simulink model "APP_Coherency_System_Rev_0_App"  (R2022b)
settings: Solver=FixedStepDiscrete  StartTime=0.0  StopTime=1  FixedStep=1e-3  MaxStep=1e-3  RelTol=1e-3
libraries: simulink x2, pil_lib x1
settings Model: Creator=HiTech  LastModifiedBy=HiTech
settings OptimizationCC: DefaultParameterBehavior=Inlined  UseDivisionForNetSlopeComputation=on  GainParamInheritBuiltInType=on  UseFloatMulNetSlope=on  InlineInvariantSignals=on  PassReuseOutputArgsAs=Individual arguments  ZeroExternalMemoryAtStartup=off  ZeroInternalMemoryAtStartup=off  NoFixptDivByZeroProtection=on  EfficientFloat2IntCast=on  LifeSpan=1  OptimizeBlockOrder=speed  DifferentSizesBufferReuse=on  EfficientTunableParamExpr=on
settings DebuggingCC: ParameterTunabilityLossMsg=error
settings HardwareCC: ProdBitPerPointer=32  ProdBitPerSizeT=32  ProdBitPerPtrDiffT=32  ProdLargestAtomicFloat=None  ProdWordSize=32  ProdLongLongMode=on  ProdHWDeviceType=Atmel->AVR (32-bit)
settings SFSimCC: MATLABDynamicMemAlloc=off
settings RTWCC: Description=Embedded Coder  SystemTargetFile=ert.tlc  TemplateMakefile=ert_default_tmf
settings CodeAppCC: ForceParamTrailComments=on  IgnoreCustomStorageClasses=off  OperatorAnnotations=on  SimulinkDataObjDesc=on  SFDataObjDesc=on  CustomSymbolStrGlobalVar=rt$N$M  CustomSymbolStrType=$N$M  CustomSymbolStrFcn=$N$M$F  CustomSymbolStrMacro=$N$M  InsertBlockDesc=on
settings ERTTargetCC: TargetLangStandard=C99 (ISO)  GenerateSampleERTMain=on  IncludeMdlTerminateFcn=off  CombineSignalStateStructs=on  SuppressErrorStatus=on  SupportAbsoluteTime=off  SupportComplex=off  InlinedParameterPlacement=NonHierarchical  ERTCustomFileTemplate=example_file_process.tlc  ERTFilePackagingFormat=CompactWithDataFile

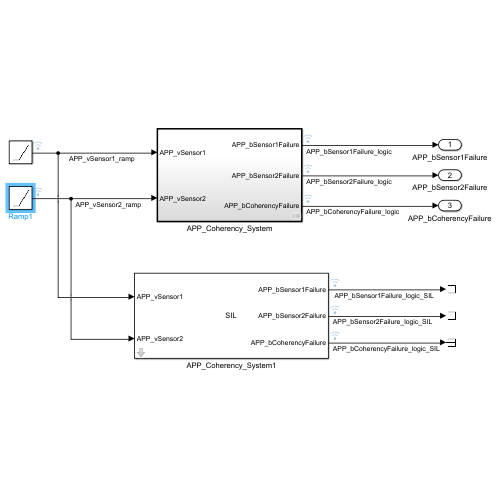
[thumbnail: Simulink's stored preview of the top-level diagram]
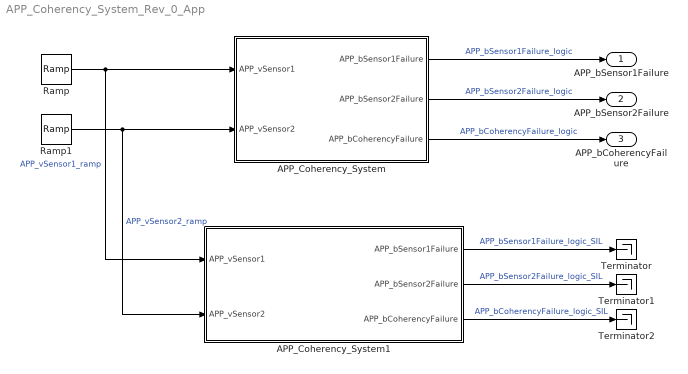
== system APP_Coherency_System_Rev_0_App ==
  APP_Coherency_System : Subsystem  TreatAsAtomicUnit=on
  APP_Coherency_System1 : Subsystem  Tag=__SL_testing_harness_stub_  DialogController=pil_create_dialog  LoadFcn=|
      | try
      |    if ~strcmp(rtw.pil.getPILVersion, '9.13 (R2022b)_15')
      |       set_param(gcb, 'DialogController', '');
      |       set_param(gcb, 'DialogControllerArgs', '');
      |    end
      | catch e
      |       set_param(gcb, 'DialogController', '');
      |       set_param(gcb, 'DialogControllerArgs', '');
      | end
      mask help: PIL:pil:XILBlockMaskDesc
      mask Display: disp('SIL');
  Ramp : simulink/Sources/Ramp  slope=4  start=0  InitialOutput=0.5
  Ramp1 : simulink/Sources/Ramp  slope=-4  start=0  InitialOutput=4.5
  Terminator : Terminator
  Terminator1 : Terminator
  Terminator2 : Terminator
  APP_bSensor1Failure : Outport
  APP_bSensor2Failure : Outport  Port=2
  APP_bCoherencyFailure : Outport  Port=3
  wires:
  APP_Coherency_System/1(APP_bSensor1Failure) -> APP_bSensor1Failure/1  "APP_bSensor1Failure_logic"
  APP_Coherency_System/2(APP_bSensor2Failure) -> APP_bSensor2Failure/1  "APP_bSensor2Failure_logic"
  APP_Coherency_System/3(APP_bCoherencyFailure) -> APP_bCoherencyFailure/1  "APP_bCoherencyFailure_logic"
  APP_Coherency_System1/1(APP_bSensor1Failure) -> Terminator/1  "APP_bSensor1Failure_logic_SIL"
  APP_Coherency_System1/2(APP_bSensor2Failure) -> Terminator1/1  "APP_bSensor2Failure_logic_SIL"
  APP_Coherency_System1/3(APP_bCoherencyFailure) -> Terminator2/1  "APP_bCoherencyFailure_logic_SIL"
  Ramp/1 -> APP_Coherency_System1/1(APP_vSensor1), APP_Coherency_System/1(APP_vSensor1)  "APP_vSensor1_ramp"
  Ramp1/1 -> APP_Coherency_System1/2(APP_vSensor2), APP_Coherency_System/2(APP_vSensor2)  "APP_vSensor2_ramp"

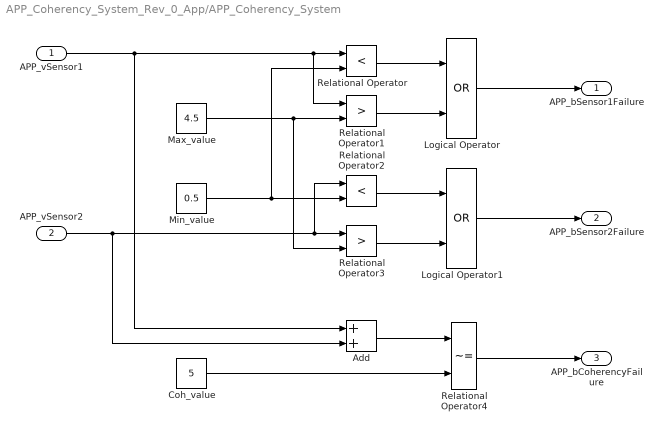
== system APP_Coherency_System_Rev_0_App/APP_Coherency_System ==
  APP_vSensor1 : Inport
  APP_vSensor2 : Inport  Port=2
  Add : Sum
  Coh_value : Constant  Value=5
  Logical Operator : Logic  Operator=OR  AllPortsSameDT=off  OutDataTypeStr=boolean
  Logical Operator1 : Logic  Operator=OR  AllPortsSameDT=off  OutDataTypeStr=boolean
  Max_value : Constant  Value=4.5
  Min_value : Constant  Value=0.5
  Relational Operator : RelationalOperator  Operator=<  OutDataTypeStr=boolean  RndMeth=Simplest  InputSameDT=off
  Relational Operator1 : RelationalOperator  Operator=>  OutDataTypeStr=boolean  RndMeth=Simplest  InputSameDT=off
  Relational Operator2 : RelationalOperator  Operator=<  OutDataTypeStr=boolean  RndMeth=Simplest  InputSameDT=off
  Relational Operator3 : RelationalOperator  Operator=>  OutDataTypeStr=boolean  RndMeth=Simplest  InputSameDT=off
  Relational Operator4 : RelationalOperator  Operator=~=  OutDataTypeStr=boolean  RndMeth=Simplest  InputSameDT=off
  APP_bSensor1Failure : Outport
  APP_bSensor2Failure : Outport  Port=2
  APP_bCoherencyFailure : Outport  Port=3
  wires:
  Logical Operator/1 -> APP_bSensor1Failure/1
  Relational Operator/1 -> Logical Operator/1
  Relational Operator1/1 -> Logical Operator/2
  Relational Operator3/1 -> Logical Operator1/2
  Relational Operator2/1 -> Logical Operator1/1
  Logical Operator1/1 -> APP_bSensor2Failure/1
  Relational Operator4/1 -> APP_bCoherencyFailure/1
  Min_value/1 -> Relational Operator/2, Relational Operator2/2
  Max_value/1 -> Relational Operator3/2, Relational Operator1/2
  APP_vSensor1/1 -> Add/1, Relational Operator1/1, Relational Operator/1
  APP_vSensor2/1 -> Add/2, Relational Operator2/1, Relational Operator3/1
  Add/1 -> Relational Operator4/1
  Coh_value/1 -> Relational Operator4/2

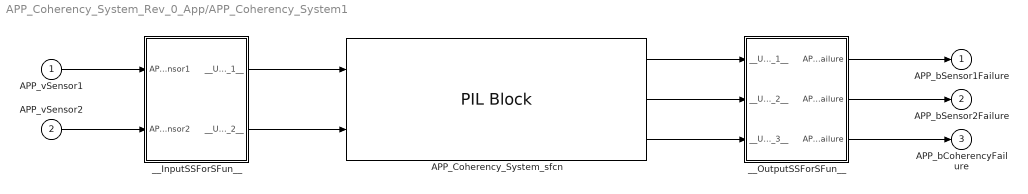
== system APP_Coherency_System_Rev_0_App/APP_Coherency_System1 ==
  APP_vSensor1 : Inport
  APP_vSensor2 : Inport  Port=2
  APP_Coherency_System_sfcn : pil_lib/PIL Block  SimulationMode=SIL  IsTopModelPIL=off  CodeDir=APP_Coherency_System_ert_rtw  AnchorDir=D:\Udemy\OS_Academy\Challenge_MAR2025\Simulink  ConfigName=Software-in-the-Loop (SIL)  XrelIsTopModelCode=on  XrelIsReusable=off  XrelDWorkNames={}  XrelDWorkTypes={}  XrelModelArgVals={}  XrelOrderedParamNames={}
  __InputSSForSFun__ : Subsystem
  __OutputSSForSFun__ : Subsystem
  APP_bSensor1Failure : Outport
  APP_bSensor2Failure : Outport  Port=2
  APP_bCoherencyFailure : Outport  Port=3
  wires:
  __OutputSSForSFun__/3(APP_bCoherencyFailure) -> APP_bCoherencyFailure/1
  __OutputSSForSFun__/2(APP_bSensor2Failure) -> APP_bSensor2Failure/1
  __OutputSSForSFun__/1(APP_bSensor1Failure) -> APP_bSensor1Failure/1
  APP_Coherency_System_sfcn/3 -> __OutputSSForSFun__/3(__UniqueInportName__3__)
  APP_Coherency_System_sfcn/2 -> __OutputSSForSFun__/2(__UniqueInportName__2__)
  APP_Coherency_System_sfcn/1 -> __OutputSSForSFun__/1(__UniqueInportName__1__)
  __InputSSForSFun__/2(__UniqueOutportName__2__) -> APP_Coherency_System_sfcn/2
  __InputSSForSFun__/1(__UniqueOutportName__1__) -> APP_Coherency_System_sfcn/1
  APP_vSensor2/1 -> __InputSSForSFun__/2(APP_vSensor2)
  APP_vSensor1/1 -> __InputSSForSFun__/1(APP_vSensor1)

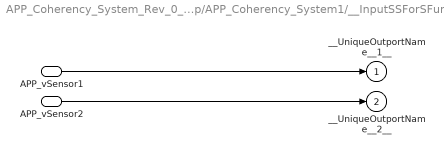
== system APP_Coherency_System_Rev_0_App/APP_Coherency_System1/__InputSSForSFun__ ==
  APP_vSensor1 : Inport
  APP_vSensor2 : Inport  Port=2
  __UniqueOutportName__1__ : Outport
  __UniqueOutportName__2__ : Outport  Port=2
  wires:
  APP_vSensor2/1 -> __UniqueOutportName__2__/1
  APP_vSensor1/1 -> __UniqueOutportName__1__/1

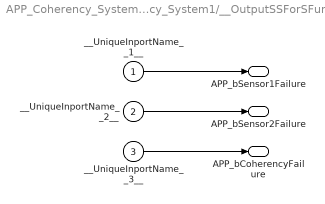
== system APP_Coherency_System_Rev_0_App/APP_Coherency_System1/__OutputSSForSFun__ ==
  __UniqueInportName__1__ : Inport
  __UniqueInportName__2__ : Inport  Port=2
  __UniqueInportName__3__ : Inport  Port=3
  APP_bSensor1Failure : Outport
  APP_bSensor2Failure : Outport  Port=2
  APP_bCoherencyFailure : Outport  Port=3
  wires:
  __UniqueInportName__3__/1 -> APP_bCoherencyFailure/1
  __UniqueInportName__2__/1 -> APP_bSensor2Failure/1
  __UniqueInportName__1__/1 -> APP_bSensor1Failure/1
